simulink model "torque_version"  (R2022a)
settings: Solver=ode15s  StartTime=0.0  StopTime=5  MaxStep=1e-2  RelTol=1e-3
values from neighbouring files (symbols this model uses):
  Disturbance_F = -100    [controller_parameters.m]
  Disturbance_S = 100    [controller_parameters.m]
  k_gn = m*g/0.01    (= 41202)    [controller_parameters.m]
  k_gt = m*g/0.01    (= 41202)    [controller_parameters.m]
  Kd = 10    [controller_parameters.m]
  Kd_pitch = 8    [controller_parameters.m]
  Kp = 100    [controller_parameters.m]
  Kp_pitch = 100    [controller_parameters.m]
  m = 42    [controller_parameters.m]    (also in ground_reaction_params.m = 12)
  m_body = m_total/2    (= 20)    [controller_parameters.m]
  m_legs = m_total/2    (= 20)    [controller_parameters.m]
  mu_slide = 0.8    [controller_parameters.m]    (also in ground_reaction_params.m = 0.008)
  mu_stick = 0.9    [controller_parameters.m]    (also in ground_reaction_params.m = 0.009)
  v_gn_max = 0.03    [controller_parameters.m]
  v_gt_max = 0.03    [controller_parameters.m]
  vLimit = 0.01    [controller_parameters.m]    (also in ground_reaction_params.m = 0.001)
undefined symbols (not defined in the file or in its folder): Newton, Raphson, X, Y, Z
libraries: sm_lib x180, nesl_utility x113, simulink x32, simulink_extras x8
(part 1 of 8)
settings Model: Creator=nemo  LastModifiedBy=prass
settings ExplorerConfigSet: InternalSimMechanicsExplorerSettings="<ExplorerConfiguration><canonicalview>default</canonicalview><AnimationSetting><BasePlaybackSpeed>1.0</BasePlaybackSpeed><PlaybackSpeedFactor>1.0</PlaybackSpeedFactor></AnimationSetting><TilePanel><TileInfo><Tiles Columns=\"2\" Count=\"4\" Rows=\"2\"><Column Weight=\"0.4995\"/><Column Weight=\"0.5005\"/><Row Weight=\"0.5011\"/><Row Weight=\"0.4989\"/><Tile Height=\"1\" Width=\"1\" X=\"0\" Y=\"0\"/><Tile Height=\"1\" Width=\"1\" X=\"0\" Y=\"1\"/><Tile Height=\"1\" Width=\"1\" X=\"1\" Y=\"0\"/><Tile Height=\"1\" Width=\"1\" X=\"1\" Y=\"1\"/></Tiles></TileInfo><SceneInfo><SceneViewer><BGColor><R>0.60000002384185791</R><G>0.60000002384185791</G><B>0.60000002384185791</B></BGColor><Camera><DoPerspective>off</DoPerspective><Position><X>1.83284282684326172e-06</X><Y>-0.997516863048076186</Y><Z>0.27808042669742733</Z></Position><Center><X>1.83284282684326172e-06</X><Y>0.00248313695192375894</Y><Z>0.27808042669742733</Z></Center><Up><X>0</X><Y>-0</Y><Z>1</Z></Up><ViewLimDist>1</ViewLimDist><YLim>0.285865645706653626</YLim><XLim>0.586843131714980593</XLim></Camera></SceneViewer><SceneViewer><BGColor><R>0.60000002384185791</R><G>0.60000002384185791</G><B>0.60000002384185791</B></BGColor><Camera><DoPerspective>off</DoPerspective><Position><X>-0.0112817941153922283</X><Y>0.0119829231240492773</Y><Z>1.27650483315918462</Z></Position><Center><X>-0.0103083985693581577</X><Y>0.00580752469879051558</Y><Z>0.276524374872420486</Z></Center><Up><X>0.00423465624963910783</X><Y>0.999971991447773156</Y><Z>-0.00617122406204799728</Z></Up><ViewLimDist>1</ViewLimDist><YLim>0.0940770085760817276</YLim><XLim>0.193981796444487098</XLim></Camera></SceneViewer><SceneViewer><BGColor><R>0.60000002384185791</R><G>0.60000002384185791</G><B>0.60000002384185791</B></BGColor><Camera><DoPerspective>off</DoPerspective><Position><X>1.00000183284282684</X><Y>0.00248314812779470984</Y><Z>0.276821106672287875</Z></Position><Center><X>1.83284282684326172e-06</X><Y>0.00248314812779470984</Y><Z>0.276821106672287875</Z></Center><Up><X>-0</X><Y>0</Y><Z>1</Z></Up><ViewLimDist>1</ViewLimDist><YLim>0.285865645706653626</YLim><XLim>0.588102451740119991</XLim></Camera></SceneViewer><SceneViewer><BGColor><R>0.60000002384185791</R><G>0.60000002384185791</G><B>0.60000002384185791</B></BGColor><Camera><DoPerspective>off</DoPerspective><Position><X>0.564257672156223467</X><Y>-0.561772691185602469</Y><Z>0.831448419529584815</Z></Position><Center><X>-0.0130925970334023756</X><Y>0.0155775780040232625</Y><Z>0.254098150339958972</Z></Center><Up><X>-0.408248290463863073</X><Y>0.408248290463863073</Y><Z>0.816496580927726145</Z></Up><ViewLimDist>1</ViewLimDist><YLim>0.276906320452690147</YLim><XLim>0.572191378988523458</XLim></Camera></SceneViewer></SceneInfo></TilePanel><MechEditorPanel><Cameras/><GfxPanelCameraMap/><VideoCreator><PlaybackSpeedRatio>1.0</PlaybackSpeedRatio><FrameRate>30</FrameRate><VideoFormat>MPEG-4</VideoFormat><FrameSize>[1920 1080]</FrameSize></VideoCreator></MechEditorPanel></ExplorerConfiguration>"

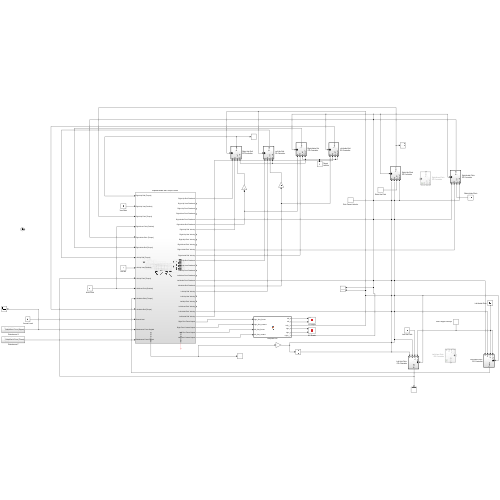
[thumbnail: Simulink's stored preview of the top-level diagram]
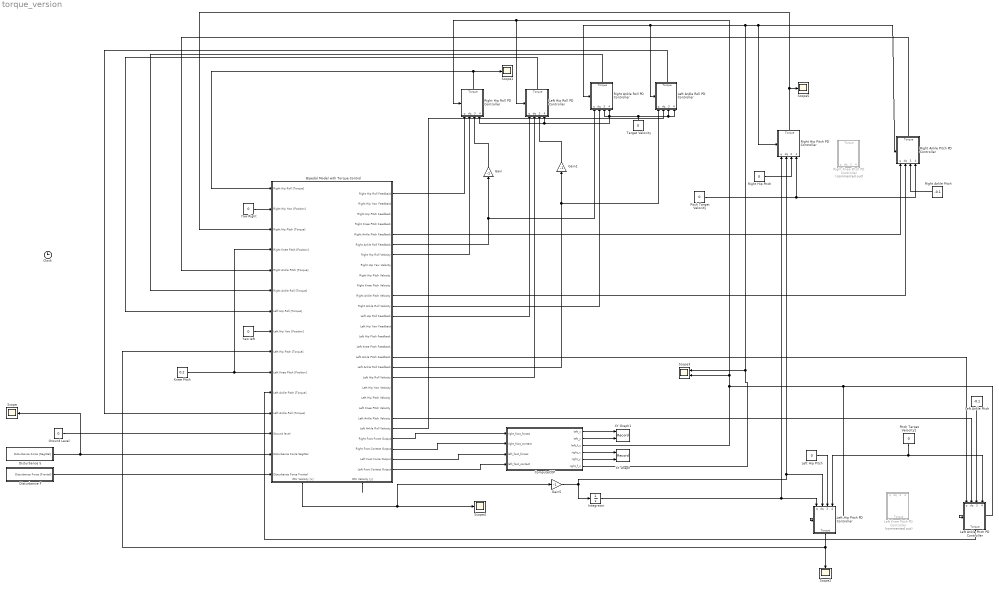
== system torque_version ==
  " Left Ankle Pitch" : Constant  Value=-0.1
  " Left Hip Pitch" : Constant  Value=0
  " Right Ankle Pitch" : Constant  Value=-0.1
  " Right Hip Pitch" : Constant  Value=0
  Bipedal Model with Torque Control : Subsystem
      settings: PortSchema="{\"entries\":[{\"content\":{\"sides\":[{\"content\":{\"connectorIds\":[\"In1\",\"In2\",\"In3\",\"In4\",\"In5\",\"In6\",\"In7\",\"In8\",\"In9\",\"In10\",\"In11\",\"In12\",\"In13\",\"In14\",\"In15\"]},\"type\":\"ConnectorPlacement.EquallySpacedRectSide\",\"uuid\":\"3dea75c4-ebd6-492f-9f7b-96a50e9bafa9\"},{\"content\":{\"connectorIds\":[\"Out1\",\"Out2\",\"Out3\",\"Out4\",\"Out5\",\"Out6\",\"Out7\",\"Out8\",\"Out9\",\"Out10\",\"Out11\",\"Out12\",\"Out13\",\"Out14\",\"Out15\",\"Out16\",\"Out17\",\"Out18\",\"Out19\",\"Out20\",\"Out21\",\"Out22\",\"Out23\",\"Out24\",\"Out25\",\"Out26\",\"Out27\",\"Out28\"],\"side\":\"RIGHT\"},\"type\":\"ConnectorPlacement.EquallySpacedRectSide\",\"uuid\":\"c9c74a48-5940-42ed-a249-f4a662242d88\"},{\"content\":{\"connectorIds\":[],\"side\":\"TOP\"},\"type\":\"ConnectorPlacement.EquallySpacedRectSide\",\"uuid\":\"1e73d28e-b625-4745-a57a-ade1903b4dfb\"},{\"content\":{\"connectorIds\":[\"Out29\",\"Out30\"],\"side\":\"BOTTOM\"},\"type\":\"ConnectorPlacement.EquallySpacedRectSide\",\"uuid\":\"8a909301-7900-4868-9293-fd81c5f76e4b\"}]},\"type\":\"ConnectorPlacement.EquallySpacedConnector\",\"uuid\":\"a749686d-b87e-4a57-b74b-aaeb9efd22c2\"}],\"packageUris\":[\"http://schema.mathworks.com/mf0/Connector/R2020b\"],\"version\":\"1.0\"}"
  Clock : Clock
  "ComputeCOP " : MATLAB Function  TreatAsAtomicUnit=on
  Disturbance F : Subsystem
  Disturbance S : Subsystem
  Gain : Gain  Gain=-1
  Gain1 : Gain  Gain=-1
  Gain5 : Gain  Gain=-1
  Ground Level : Constant  Value=0
  Integrator : Integrator
  Knee Pitch : Constant  Value=0.2
  Left Ankle Pitch PD Controller : Subsystem
  Left Ankle Roll PD Controller : Subsystem
  Left Hip Pitch PD Controller : Subsystem
  Left Hip Roll PD Controller : Subsystem
  Left Knee Pitch PD Controller : Subsystem  Commented=on
  Pitch Target Velocity : Constant  Value=0
  Pitch Target Velocity1 : Constant  Value=0
  Right Ankle Pitch PD Controller : Subsystem
  Right Ankle Roll PD Controller : Subsystem
  Right Hip Pitch PD Controller : Subsystem
  Right Hip Roll PD Controller : Subsystem
  Right Knee Pitch PD Controller : Subsystem  Commented=on
  Scope{,1..2,4..5} (5 alike) : Scope
  Scope3 : Scope  NumInputPorts=2
  Target Velocity : Constant  Value=0
  XY Graph : Record  FileSettingsInternal="{\"entries\":[{\"content\":{\"excelSettings\":{\"content\":{},\"type\":\"Streamout.ExcelSettings\"}},\"type\":\"Streamout.FileSettingStorage\",\"uuid\":\"edd4b35f-e61b-4cd1-9338-e900d54a8caa\"}],\"packageUris\":[\"http://schema.mathworks.com/mf0/streamout_blocks/R2020a\"],\"version\":\"1.0\"}"  Layout=[1 1]  SignalsInternal="{\"entries\":[{\"content\":{\"signals\":[{\"content\":{\"blockPath\":[\"torque_version/XY Graph\"],\"channel\":[],\"dimensions\":[1],\"domain\":\"torque_version/XY Graph\",\"lineColor\":\"#a2142f\",\"plots\":[1],\"port\":1,\"sid\":[],\"signalID\":17,\"signalName\":\"ComputeCOP :4\"},\"type\":\"RecordBlkView.Signal\",\"uuid\":\"83af58bc-32d3-45b1-8ec1-43a67c0f0419\"},{\"content\":{\"blockPath\":[\"torque_version/XY Graph\"],\"channel\":[],\"dimensions\":[1],\"domain\":\"torque_version/XY Graph\",\"lineColor\":\"#139fff\",\"plots\":[1],\"port\":2,\"sid\":[],\"signalID\":20,\"signalName\":\"ComputeCOP :5\"},\"type\":\"RecordBlkView.Signal\",\"uuid\":\"a9f77b6b-902b-4489-8509-e6605344718f\"}]},\"type\":\"RecordBlkView.InputSignals\",\"uuid\":\"712727bd-46d9-4345-ba5f-d59f122f9c34\"}],\"packageUris\":[\"http://schema.mathworks.com/mf0/streamout_blocks/R2020a\"],\"version\":\"1.0\"}"  VisualizationBindings="{\"xyplotplugin\":{\"info\":[{\"series\":[{\"bindingParametersList\":[{\"parameter\":\"X-Axis\",\"signalID\":17,\"signalName\":\"ComputeCOP :4\"},{\"parameter\":\"Y-Axis\",\"signalID\":20,\"signalName\":\"ComputeCOP :5\"}],\"seriesID\":3788}],\"subplotID\":1}]}}"  CompatibilityTag=XY
  XY Graph1 : Record  FileSettingsInternal="{\"entries\":[{\"content\":{\"excelSettings\":{\"content\":{},\"type\":\"Streamout.ExcelSettings\"}},\"type\":\"Streamout.FileSettingStorage\",\"uuid\":\"8acd65a4-d1fa-42fa-a465-bad077f3651d\"}],\"packageUris\":[\"http://schema.mathworks.com/mf0/streamout_blocks/R2020a\"],\"version\":\"1.0\"}"  Layout=[1 1]  SignalsInternal="{\"entries\":[{\"content\":{\"signals\":[{\"content\":{\"blockPath\":[\"torque_version/XY Graph1\"],\"channel\":[],\"dimensions\":[1],\"domain\":\"torque_version/XY Graph1\",\"lineColor\":\"#a2142f\",\"plots\":[1],\"port\":1,\"sid\":[],\"signalID\":9,\"signalName\":\"ComputeCOP :1\"},\"type\":\"RecordBlkView.Signal\",\"uuid\":\"0e1453ec-719c-4b54-9f47-88130e08b6ce\"},{\"content\":{\"blockPath\":[\"torque_version/XY Graph1\"],\"channel\":[],\"dimensions\":[1],\"domain\":\"torque_version/XY Graph1\",\"lineColor\":\"#139fff\",\"plots\":[1],\"port\":2,\"sid\":[],\"signalID\":12,\"signalName\":\"ComputeCOP :2\"},\"type\":\"RecordBlkView.Signal\",\"uuid\":\"c82dfa56-c16d-4086-ab84-ff118f72557d\"}]},\"type\":\"RecordBlkView.InputSignals\",\"uuid\":\"4dcef6cb-9ce4-4e24-874b-da2edc7d9e64\"}],\"packageUris\":[\"http://schema.mathworks.com/mf0/streamout_blocks/R2020a\"],\"version\":\"1.0\"}"  VisualizationBindings="{\"xyplotplugin\":{\"info\":[{\"series\":[{\"bindingParametersList\":[{\"parameter\":\"X-Axis\",\"signalID\":9,\"signalName\":\"ComputeCOP :1\"},{\"parameter\":\"Y-Axis\",\"signalID\":12,\"signalName\":\"ComputeCOP :2\"}],\"seriesID\":833}],\"subplotID\":1}]}}"  CompatibilityTag=XY
  Yaw Right : Constant  Value=0
  Yaw left : Constant  Value=0
  wires:
  Disturbance S/1(Disturbance Force [Sagittal]) -> Scope/1, Bipedal Model with Torque Control/14(Disturbance Force Sagittal)
  Ground Level/1 -> Bipedal Model with Torque Control/13(Ground level)
  Bipedal Model with Torque Control/25(Right Foot Force Output) -> "ComputeCOP "/1(right_foot_forces)
  Bipedal Model with Torque Control/26(Right Foot Contact Output) -> "ComputeCOP "/2(right_foot_contact)
  Bipedal Model with Torque Control/28(Left Foot Contact Output) -> "ComputeCOP "/4(left_foot_contact)
  Bipedal Model with Torque Control/27(Left Foot Force Output) -> "ComputeCOP "/3(left_foot_forces)
  Bipedal Model with Torque Control/6(Right Ankle Roll Feedback) -> Right Ankle Roll PD Controller/1(q), Gain/1
  Bipedal Model with Torque Control/12(Right Ankle Roll Velocity) -> Right Ankle Roll PD Controller/2(dq)
  Right Ankle Roll PD Controller/1(Torque) -> Bipedal Model with Torque Control/6(Right Ankle Roll [Torque])
  Bipedal Model with Torque Control/18(Left Ankle Roll Feedback) -> Left Ankle Roll PD Controller/1(q), Gain1/1
  Left Ankle Roll PD Controller/1(Torque) -> Bipedal Model with Torque Control/12(Left Ankle Roll [Torque])
  Bipedal Model with Torque Control/24(Left Ankle Roll Velocity) -> Left Ankle Roll PD Controller/2(dq)
  Target Velocity/1 -> Right Ankle Roll PD Controller/3(q_ref), Right Hip Roll PD Controller/4(dq_ref), Left Hip Roll PD Controller/4(dq_ref), Right Ankle Roll PD Controller/4(dq_ref), Left Ankle Roll PD Controller/4(dq_ref), Left Ankle Roll PD Controller/3(q_ref)
  Right Hip Roll PD Controller/1(Torque) -> Scope1/1, Bipedal Model with Torque Control/1(Right Hip Roll [Torque])
  Left Hip Roll PD Controller/1(Torque) -> Bipedal Model with Torque Control/7(Left Hip Roll [Torque])
  Bipedal Model with Torque Control/1(Right Hip Roll Feedback) -> Right Hip Roll PD Controller/1(q)
  Bipedal Model with Torque Control/7(Right Hip Roll Velocity) -> Right Hip Roll PD Controller/2(dq)
  Bipedal Model with Torque Control/13(Left Hip Roll Feedback) -> Left Hip Roll PD Controller/1(q)
  Bipedal Model with Torque Control/19(Left Hip Roll Velocity) -> Left Hip Roll PD Controller/2(dq)
  Yaw left/1 -> Bipedal Model with Torque Control/8(Left Hip Yaw [Position])
  "ComputeCOP "/3(left_f_c) -> Left Hip Pitch PD Controller/Enable, Left Ankle Pitch PD Controller/Enable, Right Hip Roll PD Controller/Enable, Left Hip Roll PD Controller/Enable, Scope3/2
  "ComputeCOP "/6(right_f_c) -> Left Ankle Roll PD Controller/Enable, Right Ankle Roll PD Controller/Enable, Right Ankle Pitch PD Controller/Enable, Right Hip Pitch PD Controller/Enable, Scope3/1
  Gain1/1 -> Left Hip Roll PD Controller/3(q_ref)
  Gain/1 -> Right Hip Roll PD Controller/3(q_ref)
  "ComputeCOP "/4(right_x) -> XY Graph/1
  "ComputeCOP "/5(right_y) -> XY Graph/2
  Yaw Right/1 -> Bipedal Model with Torque Control/2(Right Hip Yaw [Position])
  Right Ankle Pitch PD Controller/1(Torque) -> Bipedal Model with Torque Control/5(Right Ankle Pitch [Torque])
  Left Hip Pitch PD Controller/1(Torque) -> Scope2/1, Bipedal Model with Torque Control/9(Left Hip Pitch [Torque])
  Left Ankle Pitch PD Controller/1(Torque) -> Bipedal Model with Torque Control/11(Left Ankle Pitch [Torque])
  Bipedal Model with Torque Control/17(Left Ankle Pitch Feedback) -> Left Ankle Pitch PD Controller/1(q)
  Bipedal Model with Torque Control/23(Left Ankle Pitch Velocity) -> Left Ankle Pitch PD Controller/2(dq)
  Bipedal Model with Torque Control/5(Right Ankle Pitch Feedback) -> Right Ankle Pitch PD Controller/1(q)
  Bipedal Model with Torque Control/11(Right Ankle Pitch Velocity) -> Right Ankle Pitch PD Controller/2(dq)
  Pitch Target Velocity/1 -> Right Ankle Pitch PD Controller/4(dq_ref), Right Hip Pitch PD Controller/4(dq_ref)
  Pitch Target Velocity1/1 -> Left Ankle Pitch PD Controller/4(dq_ref), Left Hip Pitch PD Controller/4(dq_ref)
  " Right Ankle Pitch"/1 -> Right Ankle Pitch PD Controller/3(q_ref)
  " Left Ankle Pitch"/1 -> Left Ankle Pitch PD Controller/3(q_ref)
  " Left Hip Pitch"/1 -> Left Hip Pitch PD Controller/3(q_ref)
  " Right Hip Pitch"/1 -> Right Hip Pitch PD Controller/3(q_ref)
  Integrator/1 -> Right Hip Pitch PD Controller/1(q), Left Hip Pitch PD Controller/1(q)
  Knee Pitch/1 -> Bipedal Model with Torque Control/10(Left Knee Pitch [Position]), Bipedal Model with Torque Control/4(Right Knee Pitch [Position])
  Bipedal Model with Torque Control/29(IMU Velcoity [x]) -> Gain5/1, Scope4/1
  Gain5/1 -> Left Hip Pitch PD Controller/2(dq), Right Hip Pitch PD Controller/2(dq), Integrator/1
  Right Hip Pitch PD Controller/1(Torque) -> Scope5/1, Bipedal Model with Torque Control/3(Right Hip Pitch [Torque])
  Disturbance F/1(Disturbance Force [Frontal]) -> Bipedal Model with Torque Control/15(Disturbance Force Frontal)
  Bipedal Model with Torque Control/30(IMU Velcoity [y]) -> ?
  "ComputeCOP "/1(left_x) -> XY Graph1/1
  "ComputeCOP "/2(left_y) -> XY Graph1/2
